simulink model "clik_phi_inverse"  (R2022b)
settings: Solver=ode1  StartTime=0.0  StopTime=4  FixedStep=0.001  RelTol=1e-3
undefined symbols (not defined in the file): DiscIntNeverNeededParam, q0, Tc
settings Model: Creator=Xp  LastModifiedBy=DELL
settings SolverCC: AlgebraicLoopSolver=TrustRegion
settings DataIOCC: LimitDataPoints=on  SaveFormat=Array  SignalLoggingSaveFormat=ModelDataLogs  ReturnWorkspaceOutputs=off
settings OptimizationCC: ExpressionDepthLimit=2147483647  InitFltsAndDblsToZero=on  LifeSpan=inf
settings DebuggingCC: SaveWithParameterizedLinksMsg=none  UnderspecifiedInitializationDetection=Classic  MergeDetectMultiDrivingBlocksExec=none  SolverPrmCheckMsg=warning  MultiTaskDSMMsg=warning  MultiTaskCondExecSysMsg=none  FcnCallInpInsideContextMsg=warning  UnconnectedInputMsg=warning  UnconnectedOutputMsg=warning  UnconnectedLineMsg=warning  StateNameClashWarn=warning  SFUnexpectedBacktrackingDiag=warning  SFNoUnconditionalDefaultTransitionDiag=warning  SFExecutionAtInitializationDiag=none  SFMachineParentedDataDiag=warning  ArithmeticOperatorsInVariantConditions=warning
settings HardwareCC: ProdBitPerPointer=32  ProdBitPerSizeT=32  ProdBitPerPtrDiffT=32  ProdLargestAtomicFloat=None  ProdIntDivRoundTo=Undefined  ProdEndianess=Unspecified  ProdWordSize=32  ProdHWDeviceType=32-bit Generic
settings ModelReferenceCC: EnableRefExpFcnMdlSchedulingChecks=on  PropagateSignalLabelsOutOfModel=off
settings SFSimCC: CustomCodeUndefinedFunction=UseInterfaceOnly
settings RTWCC: DLArmComputeVersion=19.05
settings CodeAppCC: StateflowObjectComments=on
settings GRTTargetCC: TargetLangStandard=C89/C90 (ANSI)  CombineOutputUpdateFcns=off  GRTInterface=on
settings ConfigComp: CovMetricSettings=dw  CovSaveCumulativeToWorkspaceVar=on  CovSaveSingleToWorkspaceVar=on

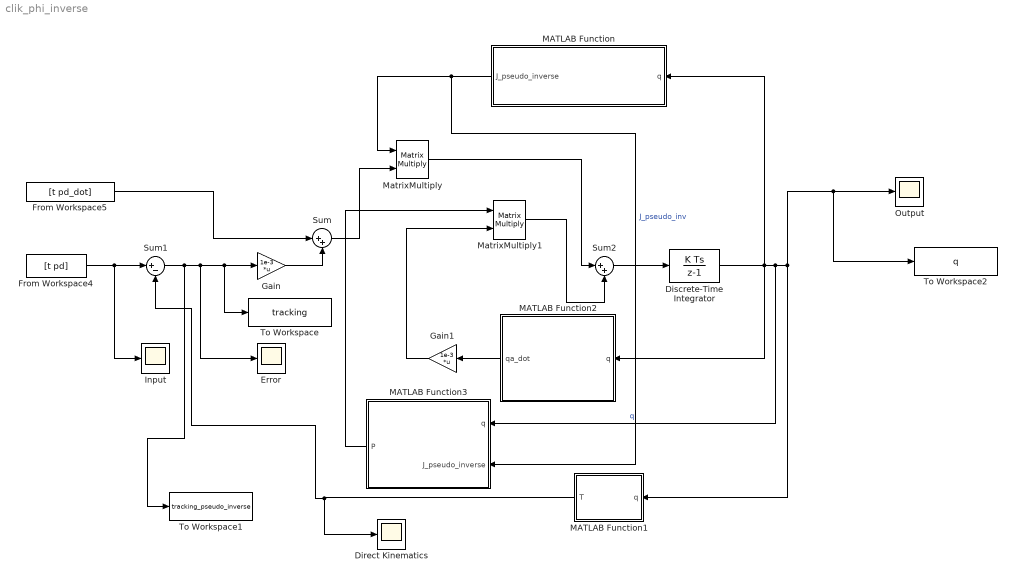
== system clik_phi_inverse ==
  Direct Kinematics : Scope
  Discrete-Time Integrator : DiscreteIntegrator  InitialCondition=q0  SampleTime=Tc  LimitOutput=on  UpperSaturationLimit=[pi/2;pi/4;1;2*pi]  LowerSaturationLimit=[-pi/2;-pi/2;0.25;-2*pi]  ICPrevOutput=DiscIntNeverNeededParam  ICPrevScaledInput=DiscIntNeverNeededParam
  Error : Scope
  From Workspace4 : FromWorkspace  VariableName=[t pd]  SampleTime=Tc
  From Workspace5 : FromWorkspace  VariableName=[t pd_dot]  SampleTime=Tc
  Gain : Gain  Gain=1e-3  Multiplication=Matrix(K*u)
  Gain1 : Gain  Gain=1e-3  Multiplication=Matrix(K*u)
  Input : Scope
  MATLAB Function : MATLAB Function  TreatAsAtomicUnit=on
  MATLAB Function1 : MATLAB Function  TreatAsAtomicUnit=on
  MATLAB Function2 : MATLAB Function  TreatAsAtomicUnit=on
  MATLAB Function3 : MATLAB Function  TreatAsAtomicUnit=on
  MatrixMultiply : Product  Multiplication=Matrix(*)
  MatrixMultiply1 : Product  Multiplication=Matrix(*)
  Output : Scope
  Sum : Sum  Inputs=|++
  Sum1 : Sum  Inputs=|+-
  Sum2 : Sum  Inputs=|++
  To Workspace : ToWorkspace  VariableName=tracking  SampleTime=Tc
  To Workspace1 : ToWorkspace  VariableName=tracking_pseudo_inverse  SampleTime=Tc
      settings: Save2DSignal=2-D array (concatenate along first dimension)
  To Workspace2 : ToWorkspace  VariableName=q  SampleTime=Tc
      settings: Save2DSignal=2-D array (concatenate along first dimension)
  wires:
  From Workspace4/1 -> Input/1, Sum1/1
  Sum1/1 -> To Workspace1/1, Error/1, Gain/1, To Workspace/1
  MATLAB Function1/1(T) -> Direct Kinematics/1, Sum1/2
  MATLAB Function/1(J_pseudo_inverse) -> MATLAB Function3/2(J_pseudo_inverse), MatrixMultiply/1  "J_pseudo_inv"
  Discrete-Time Integrator/1 -> MATLAB Function/1(q), MATLAB Function2/1(q), MATLAB Function3/1(q), MATLAB Function1/1(q), To Workspace2/1, Output/1  "q"
  Sum/1 -> MatrixMultiply/2
  From Workspace5/1 -> Sum/1
  Gain/1 -> Sum/2
  MATLAB Function2/1(qa_dot) -> Gain1/1
  MatrixMultiply/1 -> Sum2/1
  MatrixMultiply1/1 -> Sum2/2
  Sum2/1 -> Discrete-Time Integrator/1
  MATLAB Function3/1(P) -> MatrixMultiply1/1
  Gain1/1 -> MatrixMultiply1/2

== matlab function clik_phi_inverse/MATLAB Function ==
  data: q input; J_pseudo_inverse output
function J_pseudo_inverse = jacobian_pseudo_inverse(q)

% Calling the jacobian function from the jacobian matlab file
J = jacobian_phi_relax(q);

% Calculating tranpose of jacobian matrix
J_transpose = transpose(J);

JJ_transpose = J*J_transpose;

JJ_transpose_inverse = inv(JJ_transpose);

% Finally calculating pseudo-inverse of jacobian matrix
J_pseudo_inverse = J_transpose * JJ_transpose_inverse;

== matlab function clik_phi_inverse/MATLAB Function2 ==
  data: q input; qa_dot output
function qa_dot = qa_dot_function_call(q)

% Defining the maximum and minimum angle values ranges
qM = [pi/2;pi/4;1;2*pi];

qm = [-pi/2;-pi/2;0.25;-2*pi];

% Initializing qi_bar and summation
qi_bar = zeros(4,1);

summation = zeros(4,1);

for i = 1:4

    qi_bar(i) = (qM(i) + qm(i))/ 2;

    summation = summation + ((q(i) - qi_bar(i))/qM(i) - qm(i))^2;

end

w = (-1/8) * summation;

% Calculating qa_dot
qa_dot = gradient(w,q);

== matlab function clik_phi_inverse/MATLAB Function3 ==
  data: q input; P output; J_pseudo_inverse input
function P = p_matrix(q, J_pseudo_inverse)

% Calling the jacobian function from the jacobian matlab file
J = jacobian_phi_relax(q);

product = J_pseudo_inverse * J;

% Calculating the P matrix
P = eye(4,4) - product;

== matlab function clik_phi_inverse/MATLAB Function1 ==
  data: q input; T output
function T = direct_kin(q)

% Defining link length values
a1=0.5;
a2=0.5;
d0 = 1;

% Assigning individual joint values to the corresponding rows of the
% q(angle) being taken as input
q1=q(1);
q2=q(2);
d3=q(3);
q4=q(4);

% Obtained Rotation and translation direct kinematics matrix for scara manipulator
R=[cos(q1+q2+q4),sin(q1+q2+q4),0;sin(q1+q2+q4),-cos(q1+q2+q4),0;0,0,-1;0 0 0];
T=[a1*cos(q1)+a2*cos(q1+q2);a1*sin(q1)+a2*sin(q1+q2);-d3+d0];
